simulink model "q_sweep_q8_usb"  (R2014b)
settings: Solver=ode1  StartTime=0.0  StopTime=inf  FixedStep=0.0005  RelTol=1e-3
PostLoadFcn:
  | qc_set_target_type(getConfigSet(bdroot, 'QUARC Default Target Configuration'));
values from neighbouring files (symbols this model uses):
  K_AMP = 10    [config_STII.m]
  SWEEP_MAX = 4e-3    (= 0.004)    [setup.m]
  tf_sweep = 20    [setup.m]
  VMAX_AMP = Rm * IMAX_AMP    (= 44.1)    [config_STII.m]
undefined symbols (not defined in the file or in its folder): HIL, K_ENC, K_MS2G, kd, kp, qc_get_step_size
libraries: quarc_library x23, simulink x5
settings Model: SimulationMode=external  ExtModeTrigDuration=50000  Creator=MLevis  LastModifiedBy=amolki
settings SolverCC: PositivePriorityOrder=on
settings DataIOCC: SignalLoggingSaveFormat=ModelDataLogs
settings OptimizationCC: InitFltsAndDblsToZero=on
settings DebuggingCC: SaveWithParameterizedLinksMsg=none  UnderspecifiedInitializationDetection=Classic  MergeDetectMultiDrivingBlocksExec=none  MultiTaskDSMMsg=warning  MultiTaskCondExecSysMsg=none  FcnCallInpInsideContextMsg=UseLocalSettings  StateNameClashWarn=warning
settings RTWCC: SystemTargetFile=quarc_win64.tlc  TemplateMakefile=quarc_default_tmf  Description=QUARC Win64 Target  ProcessScript=quarc_win64_make_rtw_hook
settings STFCustomTargetCC: TargetPreCompLibLocation=C:\PROGRA~3\QUARC\lib\2014b\win64\release  CodeReplacementLibrary=ANSI_C  ConcurrentExecutionCompliant=on  GeneratePreprocessorConditionals=Disable all  SystemTargetFile=quarc_win64.tlc
settings GRTTargetCC: TargetPreCompLibLocation=C:\PROGRA~3\QUARC\lib\2014b\win64\release  CodeReplacementLibrary=ANSI_C  ParMdlRefBuildCompliant=off  CompOptLevelCompliant=off  CombineOutputUpdateFcns=off  MatFileLogging=off  CPPClassGenCompliant=off  GRTInterface=on  ExtMode=on  ExtModeMexFile=quarc_comm

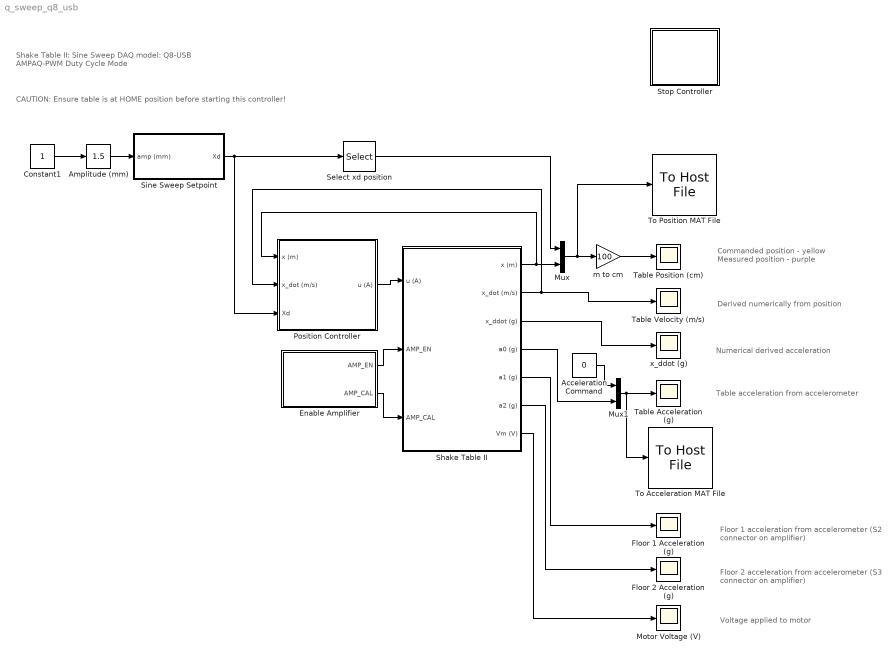
== system q_sweep_q8_usb ==
  note: Derived numerically from position
  note: Commanded position - yellow
      | Measured position - purple
  note: Numerical derived acceleration
  note: Table acceleration from accelerometer
  note: CAUTION: Ensure table is at HOME position
      | before starting this controller!
  note: Shake Table II: Sine Sweep
      | DAQ model: Q8-USB
      | AMPAQ-PWM Duty Cycle Mode
  note: Floor 2 acceleration from accelerometer
      | (S3 connector on amplifier)
  note: Floor 1 acceleration from accelerometer
      | (S2 connector on amplifier)
  note: Voltage applied to motor
  Acceleration Command : Constant  Value=0
  Amplitude (mm) : simulink/Math Operations/Slider Gain  low=0  gain=1.5  high=5
  Constant1 : Constant
  Enable Amplifier : Subsystem
  Floor 1 Acceleration (g) : Scope
      settings: TickLabels=on  TimeRange=5  YMin=-10  YMax=10  SaveName=ScopeData3
  Floor 2 Acceleration (g) : Scope
      settings: TickLabels=on  TimeRange=5  YMin=-10  YMax=10  SaveName=ScopeData6
  Motor Voltage (V) : Scope
      settings: TimeRange=25  YMin=-40  YMax=40  MaxDataPoints=25000
  Mux : Mux  Inputs=2
  Mux1 : Mux  Inputs=2
  Position Controller : Subsystem
  Select xd position : Selector  InputPortWidth=2
  "Shake Table II " : Subsystem
  Sine Sweep Setpoint : Subsystem
  Stop Controller : Subsystem
  Table Acceleration (g) : Scope
      settings: TimeRange=25  YMin=-2  YMax=2  MaxDataPoints=25000
  Table Position (cm) : Scope
      settings: TimeRange=25  YMin=-0.25  YMax=0.25  SaveName=ScopeData7  MaxDataPoints=200000
  Table Velocity (m/s) : Scope
      settings: TimeRange=25  YMin=-1  YMax=1  SaveName=ScopeData2  MaxDataPoints=25000
  To Acceleration MAT File : quarc_library/Sinks/To Host/To Host File  file_name=data_a.mat  variable_name=data_a  decimation=1  sample_time=-1  file_format=MAT-file v.4  options=No header or footer  append=off  final_file_name=data_a.mat
      settings: AttributesFormatString=%<file_name>
  To Position MAT File : quarc_library/Sinks/To Host/To Host File  file_name=data_x.mat  variable_name=data_x  decimation=1  sample_time=-1  file_format=MAT-file v.4  options=No header or footer  append=off  final_file_name=data_x.mat
      settings: AttributesFormatString=%<file_name>
  m to cm : Gain  Gain=100
  x_ddot (g) : Scope
      settings: SaveName=ScopeData5
  wires:
  Enable Amplifier/2(AMP_CAL) -> "Shake Table II "/3(AMP_CAL)
  Enable Amplifier/1("AMP_EN ") -> "Shake Table II "/2(AMP_EN)
  "Shake Table II "/2(x_dot (m/s)) -> Position Controller/2(x_dot (m/s)), Table Velocity (m/s)/1
  Sine Sweep Setpoint/1(Xd) -> Position Controller/3(Xd), Select xd position/1
  Mux/1 -> m to cm/1, To Position MAT File/1
  "Shake Table II "/5(a1 (g)) -> Floor 1 Acceleration (g)/1
  "Shake Table II "/6(a2 (g)) -> Floor 2 Acceleration (g)/1
  m to cm/1 -> Table Position (cm)/1
  "Shake Table II "/3(x_ddot (g)) -> x_ddot (g)/1
  "Shake Table II "/7(Vm (V)) -> Motor Voltage (V)/1
  Constant1/1 -> Amplitude (mm)/1
  Mux1/1 -> Table Acceleration (g)/1, To Acceleration MAT File/1
  "Shake Table II "/4(a0 (g)) -> Mux1/2
  Acceleration Command/1 -> Mux1/1
  "Shake Table II "/1(x (m)) -> Position Controller/1(x (m)), Mux/2
  Position Controller/1(u (A)) -> "Shake Table II "/1(u (A))
  Amplitude (mm)/1 -> Sine Sweep Setpoint/1(amp (mm))
  Select xd position/1 -> Mux/1

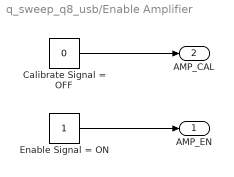
== system q_sweep_q8_usb/Enable Amplifier ==
  Calibrate Signal = OFF : Constant  Value=0  OutDataTypeStr=boolean
  Enable Signal = ON : Constant  OutDataTypeStr=boolean
  "AMP_EN " : Outport
  AMP_CAL : Outport  Port=2  InitialOutput=[0]
  wires:
  Enable Signal = ON/1 -> "AMP_EN "/1
  Calibrate Signal = OFF/1 -> AMP_CAL/1

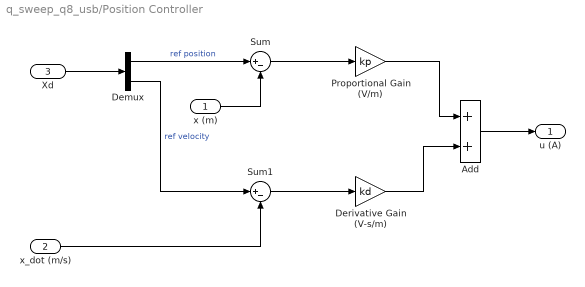
== system q_sweep_q8_usb/Position Controller ==
  x (m) : Inport
  x_dot (m/s) : Inport  Port=2
  Xd : Inport  Port=3
  Add : Sum
  Demux : Demux  Outputs=2
  Derivative Gain (V-s/m) : Gain  Gain=kd
  Proportional Gain (V/m) : Gain  Gain=kp
  Sum : Sum  Inputs=|+-
  Sum1 : Sum  Inputs=|+-
  u (A) : Outport
  wires:
  Add/1 -> u (A)/1
  Proportional Gain (V/m)/1 -> Add/1
  Derivative Gain (V-s/m)/1 -> Add/2
  Sum1/1 -> Derivative Gain (V-s/m)/1
  Sum/1 -> Proportional Gain (V/m)/1
  x_dot (m/s)/1 -> Sum1/2
  Demux/2 -> Sum1/1  "ref velocity"
  x (m)/1 -> Sum/2
  Demux/1 -> Sum/1  "ref position"
  Xd/1 -> Demux/1

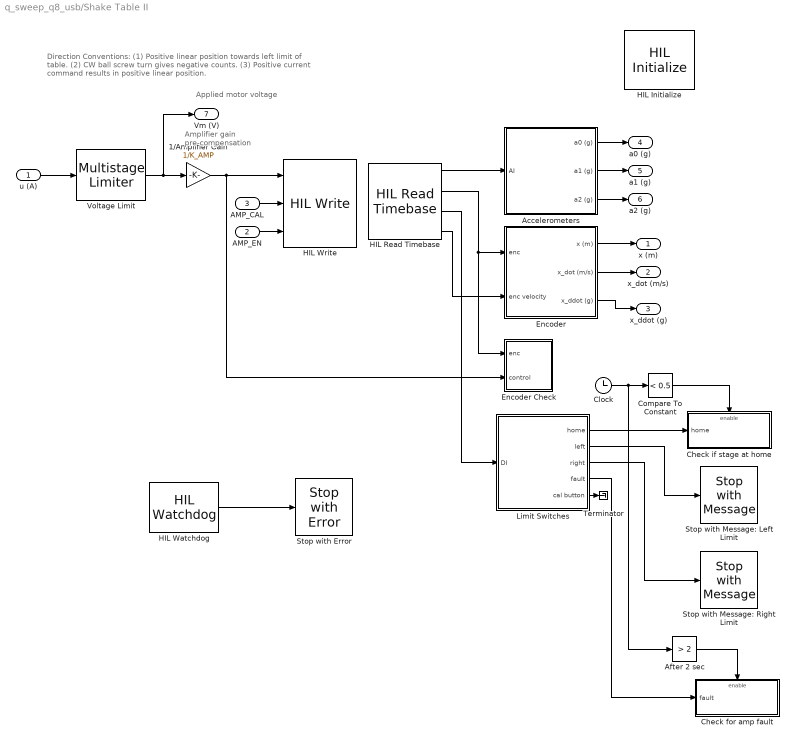
== system q_sweep_q8_usb/Shake Table II  ==
  note: Amplifier gain
      | pre-compensation
  note: Applied motor voltage
  note: Direction Conventions:
      | (1) Positive linear position towards left limit of table.
      | (2) CW ball screw turn gives negative counts.
      | (3) Positive current command results in positive linear position.
  u (A) : Inport
  AMP_EN : Inport  Port=2
  AMP_CAL : Inport  Port=3
  1/Amplifier Gain : Gain  Gain=1/K_AMP
  Accelerometers : Subsystem  Description=Accelerometer Module
  After 2 sec : simulink/Logic and Bit Operations/Compare To Constant  relop=>  const=2  OutDataTypeStr=uint8  ZeroCross=off
  Check for amp fault : Subsystem  TreatAsAtomicUnit=on
  Check if stage at home : Subsystem  TreatAsAtomicUnit=on
  Clock : Clock
  Compare To Constant : simulink/Logic and Bit Operations/Compare To Constant  relop=<  const=0.5  OutDataTypeStr=uint8  ZeroCross=off
  Encoder : Subsystem
  Encoder Check : Subsystem
  HIL Initialize : quarc_library/Data Acquisition/Generic/Configuration/HIL Initialize  object_name=HIL-1  board_type=q8_usb  board_number=0  board_options=update_rate=fast;ext_int_polarity=0;convert_polarity=1;watchdog_polarity=0;ext_int_watchdog=0;use_convert=0;pwm_immediate=0;decimation=1  exclusive=off  active=on  hardware_clocks=[0:2]  clock_modes=[]  initial_clock_frequencies=[]  set_clock_params_at_start=off  set_clock_params_at_switch_in=off  set_clock_frequencies_at_start=off  set_clock_frequencies_at_switch_in=off  analog_input_channels=[0:7]  analog_input_maximums=10  analog_input_minimums=-10  set_analog_input_params_at_start=on  set_analog_input_params_at_switch_in=off  analog_output_channels=[0:7]  analog_output_maximums=10  analog_output_minimums=-10  initial_analog_outputs=[0]  final_analog_outputs=[0]  watchdog_analog_outputs=0  set_analog_output_params_at_start=on  set_analog_output_params_at_switch_in=off  set_analog_outputs_at_start=on  set_analog_outputs_at_switch_in=off  set_analog_outputs_at_terminate=on  set_analog_outputs_at_switch_out=off  set_analog_outputs_on_watchdog=on  digital_input_channels=[0:4]  digital_output_channels=[0:7]  digital_output_configuration=[]  initial_digital_outputs=[0]  final_digital_outputs=[0]  watchdog_digital_outputs=[0]  set_digital_output_params_at_start=off  set_digital_output_params_at_switch_in=off  set_digital_outputs_at_start=on  set_digital_outputs_at_switch_in=off  set_digital_outputs_at_terminate=on  set_digital_outputs_at_switch_out=off  set_digital_outputs_on_watchdog=on  encoder_channels=[0:7]  quadrature=[4]  encoder_filter_frequency=[]  initial_encoder_counts=[0]  set_encoder_params_at_start=on  set_encoder_params_at_switch_in=off  set_encoder_counts_at_start=on  set_encoder_counts_at_switch_in=off  pwm_channels=[0:7]  pwm_modes=0  pwm_frequency=99.532799999999995e6/4095  pwm_configuration=[0]  pwm_alignment=[0]  pwm_polarity=[1]  pwm_leading_deadband=[0]  pwm_trailing_deadband=[0]  initial_pwm_outputs=[0]  final_pwm_outputs=[0]  watchdog_pwm_outputs=[0]  set_pwm_params_at_start=on  set_pwm_params_at_switch_in=off  set_pwm_outputs_at_start=on  set_pwm_outputs_at_switch_in=off  set_pwm_outputs_at_terminate=on  set_pwm_outputs_at_switch_out=off  set_pwm_outputs_on_watchdog=off  other_output_channels=[]  initial_other_outputs=[]  final_other_outputs=[]  watchdog_other_outputs=[]  set_other_outputs_at_start=off  set_other_outputs_at_switch_in=off  set_other_outputs_at_terminate=off  set_other_outputs_at_switch_out=off  set_other_outputs_on_watchdog=off
  HIL Read Timebase : quarc_library/Data Acquisition/Generic/Timebases/HIL Read Timebase  object_name=HIL-1  clock=0  analog_channels=[0:2]  encoder_channels=[0]  digital_channels=[0:4]  other_channels=[14000]  samples_in_buffer=max(ceil(1/qc_get_step_size), 1)  active=on  vector_output=on  data_type_mode=Inherit via back propagation  encoder_data_type=double  digital_data_type=boolean
  HIL Watchdog : quarc_library/Data Acquisition/Generic/Watchdog/HIL Watchdog  object_name=HIL-1  timeout=5*qc_get_step_size  sample_time=qc_get_step_size  active=off
      settings: AttributesFormatString=(%<object_name>)
  HIL Write : quarc_library/Data Acquisition/Generic/Immediate I//O/HIL Write  object_name=HIL-1  analog_channels=[0]  pwm_channels=[]  digital_channels=[0:1]  other_channels=[]  sample_time=-1  active=off  vector_input=off
  Limit Switches : Subsystem
  Stop with Error : quarc_library/Sinks/Error Handling/Stop with Error  message_type=Fixed error message  message=Stopped by Watchdog - controller began running too slow.
      settings: AttributesFormatString="\"%<message>\""
  Stop with Message: Left Limit : quarc_library/Sinks/Error Handling/Stop with Message  message_type=Fixed error message  message_icon=Error  message=Left limit switch has been triggered!
  Stop with Message: Right Limit : quarc_library/Sinks/Error Handling/Stop with Message  message_type=Fixed error message  message_icon=Error  message=Right limit switch has been triggered!
  Terminator : Terminator
  Voltage Limit : quarc_library/Discontinuities/Multistage Limiter  peak_lim=VMAX_AMP  peak_time_lim=2  cont_lim=VMAX_AMP/2  cont_hold_time=1
  x (m) : Outport  InitialOutput=0
  x_dot (m/s) : Outport  Port=2  InitialOutput=0
  x_ddot (g) : Outport  Port=3  InitialOutput=0
  a0 (g) : Outport  Port=4  InitialOutput=0
  a1 (g) : Outport  Port=5  InitialOutput=0
  a2 (g) : Outport  Port=6  InitialOutput=0
  Vm (V) : Outport  Port=7  InitialOutput=0
  wires:
  Limit Switches/1(home) -> Check if stage at home/1(home)
  Clock/1 -> Compare To Constant/1, After 2 sec/1
  Encoder/1(x (m)) -> x (m)/1
  HIL Read Timebase/3 -> Limit Switches/1(DI)
  HIL Read Timebase/1 -> Accelerometers/1(AI)
  AMP_EN/1 -> HIL Write/3
  AMP_CAL/1 -> HIL Write/2
  Limit Switches/3(right) -> Stop with Message: Right Limit/1
  Limit Switches/2(left) -> Stop with Message: Left Limit/1
  HIL Read Timebase/2 -> Encoder Check/1(enc), Encoder/1(enc)
  u (A)/1 -> Voltage Limit/1
  Accelerometers/1(a0 (g)) -> a0 (g)/1
  Accelerometers/2(a1 (g)) -> a1 (g)/1
  Accelerometers/3(a2 (g)) -> a2 (g)/1
  Compare To Constant/1 -> Check if stage at home/Enable
  Limit Switches/5(cal button) -> Terminator/1
  After 2 sec/1 -> Check for amp fault/Enable
  Limit Switches/4(fault) -> Check for amp fault/1(fault)
  HIL Watchdog/1 -> Stop with Error/1
  Encoder/3(x_ddot (g)) -> x_ddot (g)/1
  Voltage Limit/1 -> Vm (V)/1, 1/Amplifier Gain/1
  1/Amplifier Gain/1 -> Encoder Check/2(control), HIL Write/1
  Encoder/2(x_dot (m/s)) -> x_dot (m/s)/1
  HIL Read Timebase/4 -> Encoder/2(enc velocity)

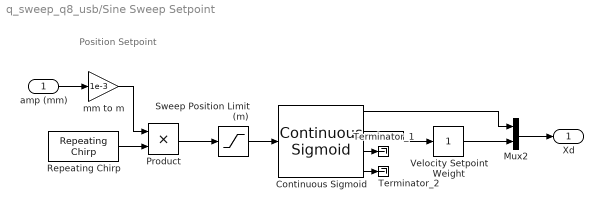
== system q_sweep_q8_usb/Sine Sweep Setpoint ==
  note: Position Setpoint
  amp (mm) : Inport
  Continuous Sigmoid : quarc_library/Sources/Sigmoids/Continuous Sigmoid  params_source=Internal (dialog parameters)  max_velocity=VEL_MAX  max_acceleration=ACC_MAX  initial_position=0  initial_velocity=0  hold_off=0.1  input_sample_time=-1  output_sample_time=qc_get_step_size
  Mux2 : Mux  Inputs=2
  Product : Product  RndMeth=Zero
  Repeating Chirp : quarc_library/Sources/Signals/Repeating Chirp  Description=Special Chirsp . starts and stops with zero...  A=1  f1=1  T=tf_sweep  f2=10  D=1
  Sweep Position Limit (m) : Saturate  UpperLimit=SWEEP_MAX  LowerLimit=-SWEEP_MAX
  Terminator_1 : Terminator
  Terminator_2 : Terminator
  Velocity Setpoint Weight : simulink/Math Operations/Slider Gain  low=0  gain=1  high=1
  mm to m : Gain  Gain=1e-3
  Xd : Outport
  wires:
  Continuous Sigmoid/4 -> Terminator_2/1
  Product/1 -> Sweep Position Limit (m)/1
  Continuous Sigmoid/1 -> Mux2/1
  Continuous Sigmoid/2 -> Velocity Setpoint Weight/1
  Velocity Setpoint Weight/1 -> Mux2/2
  Mux2/1 -> Xd/1
  Sweep Position Limit (m)/1 -> Continuous Sigmoid/1
  amp (mm)/1 -> mm to m/1
  mm to m/1 -> Product/1
  Repeating Chirp/1 -> Product/2
  Continuous Sigmoid/3 -> Terminator_1/1

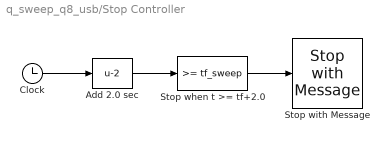
== system q_sweep_q8_usb/Stop Controller ==
  Add 2.0 sec : Bias  Bias=-2
  Clock : Clock
  Stop when t >= tf+2.0 : simulink/Logic and Bit Operations/Compare To Constant  relop=>=  const=tf_sweep  OutDataTypeStr=boolean  ZeroCross=off
  Stop with Message : quarc_library/Sinks/Error Handling/Stop with Message  message_type=Fixed error message  message_icon=Information  message=Controller finished.
  wires:
  Stop when t >= tf+2.0/1 -> Stop with Message/1
  Add 2.0 sec/1 -> Stop when t >= tf+2.0/1
  Clock/1 -> Add 2.0 sec/1

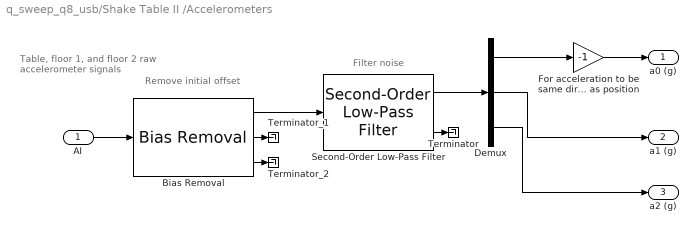
== system q_sweep_q8_usb/Shake Table II /Accelerometers ==
  note: Filter noise
  note: Remove initial offset
  note: Table, floor 1, and floor 2 raw accelerometer signals
  AI : Inport
  Bias Removal : quarc_library/Discrete/Bias Removal  start_time=0  end_time=0.1  switch_id=0  sample_time=qc_get_step_size
  Demux : Demux  Outputs=3
  For acceleration to be same direction as position : Gain  Gain=-1
  Second-Order Low-Pass Filter : quarc_library/Continuous/Second-Order Low-Pass Filter  params_source=Internal (dialog parameters)  input_width=wa  input_zeta=za  input_init=0
  Terminator : Terminator
  Terminator_1 : Terminator
  Terminator_2 : Terminator
  a0 (g) : Outport  InitialOutput=0
  a1 (g) : Outport  Port=2  InitialOutput=0
  a2 (g) : Outport  Port=3  InitialOutput=0
  wires:
  Bias Removal/2 -> Terminator_1/1
  Bias Removal/3 -> Terminator_2/1
  AI/1 -> Bias Removal/1
  For acceleration to be same direction as position/1 -> a0 (g)/1
  Demux/1 -> For acceleration to be same direction as position/1
  Demux/2 -> a1 (g)/1
  Demux/3 -> a2 (g)/1
  Bias Removal/1 -> Second-Order Low-Pass Filter/1
  Second-Order Low-Pass Filter/1 -> Demux/1
  Second-Order Low-Pass Filter/2 -> Terminator/1

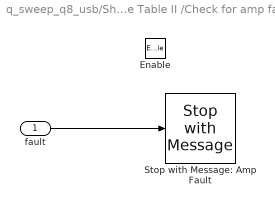
== system q_sweep_q8_usb/Shake Table II /Check for amp fault ==
  fault : Inport
  Enable : EnablePort
  Stop with Message: Amp Fault : quarc_library/Sinks/Error Handling/Stop with Message  message_type=Fixed error message  message_icon=Error  message=AMPAQ-PWM fault.
  wires:
  fault/1 -> Stop with Message: Amp Fault/1

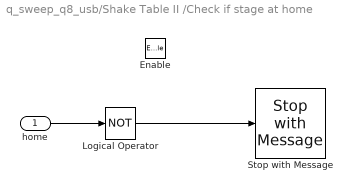
== system q_sweep_q8_usb/Shake Table II /Check if stage at home ==
  home : Inport
  Enable : EnablePort
  Logical Operator : Logic  Operator=NOT  AllPortsSameDT=off  OutDataTypeStr=boolean
  Stop with Message : quarc_library/Sinks/Error Handling/Stop with Message  message_type=Fixed error message  message_icon=Error  message=Error Table not at home. Calibrate table before starting this controller.
  wires:
  home/1 -> Logical Operator/1
  Logical Operator/1 -> Stop with Message/1

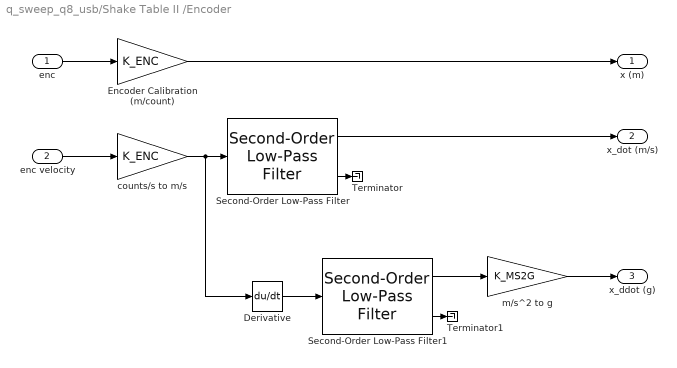
== system q_sweep_q8_usb/Shake Table II /Encoder ==
  enc : Inport
  enc velocity : Inport  Port=2
  Derivative : Derivative
  Encoder Calibration (m/count) : Gain  Gain=K_ENC  SaturateOnIntegerOverflow=on  OutDataTypeStr=Inherit: Same as input  ParamDataTypeStr=Inherit: Same as input
  Second-Order Low-Pass Filter : quarc_library/Continuous/Second-Order Low-Pass Filter  params_source=Internal (dialog parameters)  input_width=wd  input_zeta=zd  input_init=0
  Second-Order Low-Pass Filter1 : quarc_library/Continuous/Second-Order Low-Pass Filter  params_source=Internal (dialog parameters)  input_width=wa  input_zeta=za  input_init=0
  Terminator : Terminator
  Terminator1 : Terminator
  counts/s to m/s : Gain  Gain=K_ENC  SaturateOnIntegerOverflow=on  OutDataTypeStr=Inherit: Same as input  ParamDataTypeStr=Inherit: Same as input
  m/s^2 to g : Gain  Gain=K_MS2G
  x (m) : Outport  InitialOutput=0
  x_dot (m/s) : Outport  Port=2  InitialOutput=0
  x_ddot (g) : Outport  Port=3  InitialOutput=0
  wires:
  enc/1 -> Encoder Calibration (m/count)/1
  Encoder Calibration (m/count)/1 -> x (m)/1
  Derivative/1 -> Second-Order Low-Pass Filter1/1
  enc velocity/1 -> counts/s to m/s/1
  counts/s to m/s/1 -> Second-Order Low-Pass Filter/1, Derivative/1
  Second-Order Low-Pass Filter1/1 -> m/s^2 to g/1
  Second-Order Low-Pass Filter/2 -> Terminator/1
  Second-Order Low-Pass Filter1/2 -> Terminator1/1
  Second-Order Low-Pass Filter/1 -> x_dot (m/s)/1
  m/s^2 to g/1 -> x_ddot (g)/1

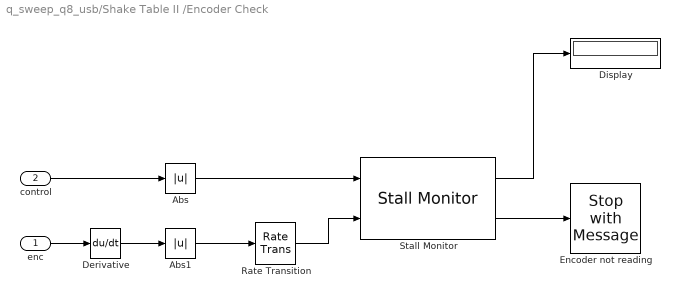
== system q_sweep_q8_usb/Shake Table II /Encoder Check ==
  enc : Inport
  control : Inport  Port=2
  Abs : Abs
  Abs1 : Abs
  Derivative : Derivative
  Display : Display
  Encoder not reading : quarc_library/Sinks/Error Handling/Stop with Message  message_type=Fixed error message  message_icon=Error  message=Current applied and not reading position. Check E-Stop and verify encoder is working.
  Rate Transition : RateTransition
  Stall Monitor : quarc_library/Discrete/Stall Monitor  control_threshold=0.5  motion_threshold=5  duration_s=0.05
  wires:
  Stall Monitor/1 -> Display/1
  Rate Transition/1 -> Stall Monitor/2
  Abs1/1 -> Rate Transition/1
  Derivative/1 -> Abs1/1
  enc/1 -> Derivative/1
  Stall Monitor/2 -> Encoder not reading/1
  control/1 -> Abs/1
  Abs/1 -> Stall Monitor/1

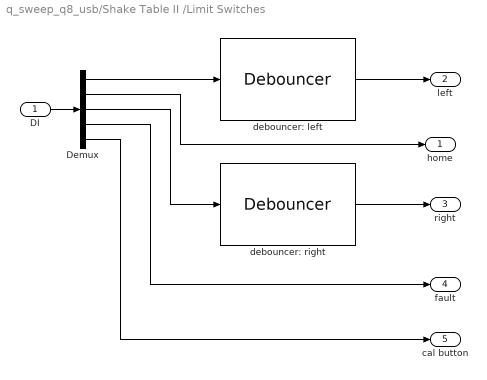
== system q_sweep_q8_usb/Shake Table II /Limit Switches ==
  DI : Inport
  Demux : Demux  Outputs=5
  debouncer: left : quarc_library/Discontinuities/Debouncer  init_state=Off  param_src=Specify via dialog  threshold=dbnc_threshold  rise_time=dbnc_rise_time  fall_time=0
  debouncer: right : quarc_library/Discontinuities/Debouncer  init_state=Off  param_src=Specify via dialog  threshold=dbnc_threshold  rise_time=dbnc_rise_time  fall_time=0
  home : Outport
  left : Outport  Port=2
  right : Outport  Port=3
  fault : Outport  Port=4
  cal button : Outport  Port=5
  wires:
  debouncer: left/1 -> left/1
  Demux/1 -> debouncer: left/1
  Demux/4 -> fault/1
  Demux/2 -> home/1
  DI/1 -> Demux/1
  Demux/3 -> debouncer: right/1
  debouncer: right/1 -> right/1
  Demux/5 -> cal button/1
